simulink model "abl_M4_rigidPPC"  (R2023b)
settings: Solver=ode45  StartTime=0.0  StopTime=80  MaxStep=1e-3  RelTol=5e-5
model workspace (MAT data in the model file):
  gpsid1 : Simulink.Signal (value not decoded)
  gpsid2 : Simulink.Signal (value not decoded)
  gpsid3 : Simulink.Signal (value not decoded)
  kkk1 : Simulink.Signal (value not decoded)
  kkk2 : Simulink.Signal (value not decoded)
  kkk3 : Simulink.Signal (value not decoded)
  psid = 0.5
undefined symbols (not defined in the file): A_raw1, A_raw2, beta1, beta2, p00, p_d_10, p_d_20, p_d_30, p_d_40, p_d_50, p_d_60, p_hat_p10, p_hat_p20, p_hat_p30, p_hat_p40, p_hat_p50, p_hat_p60, p_hat_v10, p_hat_v20, p_hat_v30, p_hat_v40, p_hat_v50, p_hat_v60, p_off_set1, p_off_set2, v00
(part 4 of 4)

== matlab function abl_M4_rigidPPC/Subsystem18/Subsystem/Guidence ==
  settings: updateMethod=DISCRETE
  data: t input; x input; y input; desire input; psi input; psid output; psi_e output; rhoe output; xd output; yd output
function [psid,psi_e,rhoe,xd,yd]  = desire(t,x,y,desire,psi)
xd = desire(1);yd = desire(4);
dxd = desire(2); dyd=desire(5);
xe =x-xd;
ye =y-yd;
 rhoe = sqrt((xe)^2+(ye)^2); 
 persistent kkk2 gpsid2
% if abs(rhoe)<1
    p = atan2(10000*ye+10*dyd,10000*xe+10*dxd);
    % u1 = 0.1*dxd+10*xe;
    % u2 = 0.1*dyd+10*ye;
    % z=u1+u2*i;
    % p=angle(z);
% else
%     p = atan2(ye,xe);
% end

if isempty(kkk2)
    kkk2=0;
    gpsid2=p;
end
if p*gpsid2<-0.7*pi^2 && p>0  %Change nearly in -pi and +pi
   kkk2=kkk2-1;
end
if p*gpsid2<-0.7*pi^2 && p<0  %Change nearly in -pi and +pi
   kkk2=kkk2+1;
end
gpsid2=p;
psid=p+2*kkk2*pi;
psi_e = psi-psid;
 
 

end

== matlab function abl_M4_rigidPPC/Subsystem18/Subsystem1/MATLAB Function1 ==
  data: x1 input; dotx1 output; dotx2 output; x2 input; psid input
function [dotx1,dotx2] = desire(x1,x2,psid)
    R  = 1;
    dotx1 = x2;
    dotx2 = -2*R^2*(x1-psid)-R*x2;
end

== matlab function abl_M4_rigidPPC/Subsystem18/Subsystem1/MATLAB Function2 ==
  data: x1 input; dotx1 output; dotx2 output; x2 input; psid input
function [dotx1,dotx2] = desire(x1,x2,psid)
    R  = 1;
    dotx1 = x2;
    dotx2 = -2*R^2*(x1-psid)-R*x2;
end

== matlab function abl_M4_rigidPPC/USV8/MATLAB Function ==
  data: t input; tau_u input; x_dot output; y_dot output; psi_dot output; u_dot output; v_dot output; r_dot output; tau_r input; psi input; u input; v input; r input
function [x_dot, y_dot, psi_dot, u_dot, v_dot, r_dot] = dynamics(t,tau_u,tau_r,psi,u, v, r)
    m11=24.9;m22=33.8;m33=2.86;
    Du=12;Dv=17;Dr=0.5;
    % Kinematic equations
    x_dot = u * cos(psi) - v * sin(psi);
    y_dot = u * sin(psi) + v * cos(psi);    
    psi_dot = r;
    % Disturbence
    tau_wu = 0.50*sin(0.1*t);
    tau_wv = 0.50*cos(0.1*t); 
    tau_wr = 0.50*sin(0.2*t);
    % Dynamic equations
    u_dot = (m22 * v * r - Du * u + tau_u + tau_wu) / m11;
    v_dot = (-m11 * u * r - Dv * v + tau_wv) / m22;
    r_dot = ((m11 - m22) * u * v - Dr * r + tau_r + tau_wr) / m33;
    % 质量和惯性参数
   

end

== matlab function abl_M4_rigidPPC/USV9/MATLAB Function ==
  data: t input; tau_u input; x_dot output; y_dot output; psi_dot output; u_dot output; v_dot output; r_dot output; tau_r input; psi input; u input; v input; r input
function [x_dot, y_dot, psi_dot, u_dot, v_dot, r_dot] = dynamics(t,tau_u,tau_r,psi,u, v, r)
    m11=24.9;m22=33.8;m33=2.86;
    Du=12;Dv=17;Dr=0.5;
    % Kinematic equations
    x_dot = u * cos(psi) - v * sin(psi);
    y_dot = u * sin(psi) + v * cos(psi);    
    psi_dot = r;
    % Disturbence
    tau_wu = 0.50*sin(0.1*t);
    tau_wv = 0.50*cos(0.1*t); 
    tau_wr = 0.50*sin(0.2*t);
    % Dynamic equations
    u_dot = (m22 * v * r - Du * u + tau_u + tau_wu) / m11;
    v_dot = (-m11 * u * r - Dv * v + tau_wv) / m22;
    r_dot = ((m11 - m22) * u * v - Dr * r + tau_r + tau_wr) / m33;
    % 质量和惯性参数
   

end
